simulink model "STM32Nucleo_VL53L1A1"  (R2023a)
settings: Solver=FixedStepDiscrete  StartTime=0.0  StopTime=inf  FixedStep=0.01  RelTol=1e-3  EnableMultiTasking=on
libraries: instrumentseriallib x3, nucleoutilitieslib x3, stmutilitieslib x3
settings Model: SimulationMode=external  PacingRate=0.100000  ExtModeTrigDuration=10  Creator=JesseJabezArendse  LastModifiedBy=JesseJabezArendse
settings OptimizationCC: ReuseModelBlockBuffer=off  PassReuseOutputArgsAs=Individual arguments  ZeroExternalMemoryAtStartup=off  ZeroInternalMemoryAtStartup=off  MaxStackSize=64  OptimizationLevel=level1  OptimizationCustomize=off  EfficientTunableParamExpr=on
settings DebuggingCC: ParameterPrecisionLossMsg=none  ParameterTunabilityLossMsg=error
settings HardwareCC: ProdBitPerPointer=32  ProdBitPerSizeT=32  ProdBitPerPtrDiffT=32  ProdLargestAtomicInteger=Long  ProdLargestAtomicFloat=Double  ProdWordSize=32  ProdLongLongMode=on  ProdHWDeviceType=ARM Compatible->ARM Cortex
settings ModelReferenceCC: EnableParallelModelReferenceBuilds=on
settings SFSimCC: SimCustomHeaderCode="#include \"Core\\Inc\\main.h\""  SimParseCustomCode=off  MATLABDynamicMemAlloc=off  SimHardwareAcceleration=native
settings SFSimCC: SimUserSources=|
  | Core\Src\main.c
  | Core\Src\IKS02A1_Simulink.c
settings SFSimCC: SimUserIncludeDirs=|
  | Core\Inc\
  | Core\Src\
settings RTWCC: Description=Embedded Coder  SystemTargetFile=ert.tlc  HardwareBoard=STM32 Nucleo F411RE  TemplateMakefile=ert_default_tmf  RTWUseSimCustomCode=on  CustomHeaderCode="#include \"Core\\Inc\\main.h\""  Toolchain=GNU Tools for ARM Embedded Processors  BuildConfiguration=Specify
settings RTWCC: CustomInclude=|
  | Core\Inc\
  | Core\Src\
settings RTWCC: CustomSource=|
  | Core\Src\main.c
  | Core\Src\IKS02A1_Simulink.c
settings CodeAppCC: ForceParamTrailComments=on  IgnoreCustomStorageClasses=off  OperatorAnnotations=on  SimulinkDataObjDesc=on  SFDataObjDesc=on  InsertBlockDesc=on
settings ERTTargetCC: CodeReplacementLibrary=ARM Cortex-M  SupportContinuousTime=on  ExtModeTransport=3  ExtModeStaticAlloc=on  ExtModeStaticAllocSize=2000  ExtModeMexFile=ext_xcp  ExtModeIntrfLevel=Level2 - Open

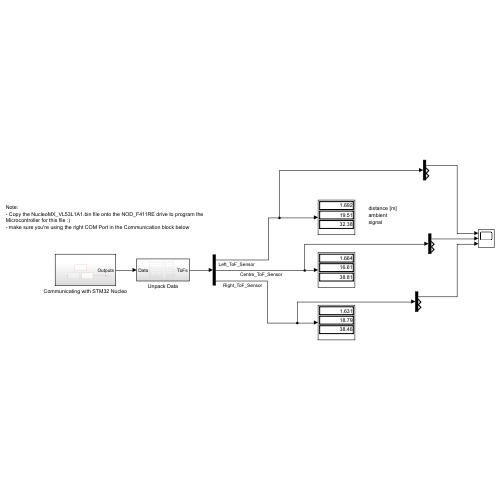
[thumbnail: Simulink's stored preview of the top-level diagram]
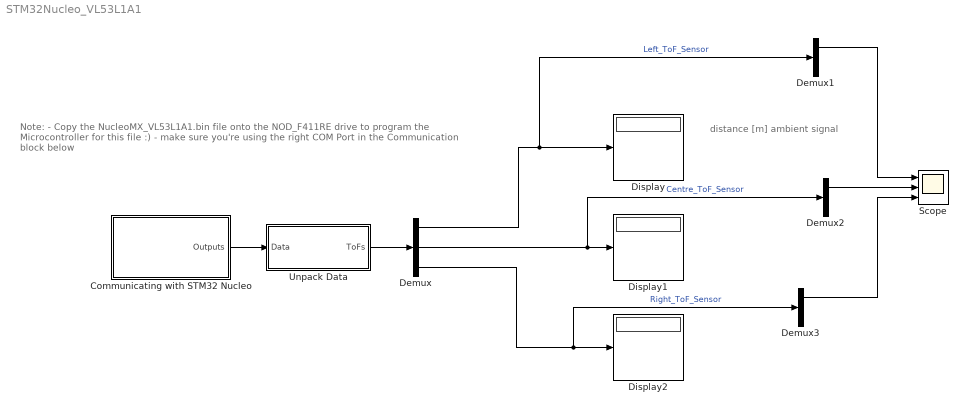
== system STM32Nucleo_VL53L1A1 ==
  note: distance [m]
      | ambient
      | signal
  note: Note:
      | - Copy the NucleoMX_VL53L1A1.bin file onto the NOD_F411RE drive to program the Microcontroller for this file :)
      | - make sure you're using the right COM Port in the Communication block below
  Communicating with STM32 Nucleo : Subsystem
  Demux : Demux  Outputs=[3 3 3]
  Demux1 : Demux  Outputs=3
  Demux2 : Demux  Outputs=3
  Demux3 : Demux  Outputs=3
  Display : Display
  Display1 : Display
  Display2 : Display
  Scope : Scope  NumInputPorts=3
  Unpack Data : Subsystem
  wires:
  Unpack Data/1(ToFs) -> Demux/1
  Demux/1 -> Demux1/1, Display/1  "Left_ToF_Sensor"
  Demux/2 -> Demux2/1, Display1/1  "Centre_ToF_Sensor"
  Demux/3 -> Demux3/1, Display2/1  "Right_ToF_Sensor"
  Communicating with STM32 Nucleo/1(Outputs) -> Unpack Data/1(Data)
  Demux1/1 -> Scope/1
  Demux2/1 -> Scope/2
  Demux3/1 -> Scope/3

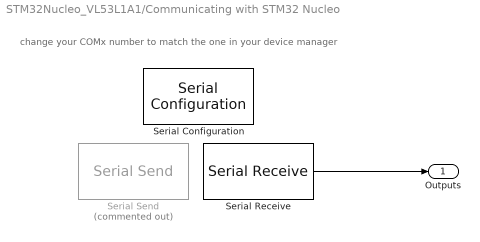
== system STM32Nucleo_VL53L1A1/Communicating with STM32 Nucleo ==
  note: change your COMx number to match the one in your device manager
  Serial Configuration : instrumentseriallib/Serial Configuration  Priority=-200000  PortSel=COM5  Port=COM5  ComPort=COM5  BaudRate=38400  DataBits=8  Parity=none  StopBits=1  ByteOrder=little-endian  FlowControl=none  Timeout=10  SimulateUsing=Interpreted execution  BlockInModel=on  aMode=1
      settings: LibrarySourceBlock=embeddedtargetslib/Host Communication/Serial Configuration
  Serial Receive : instrumentseriallib/Serial Receive  Priority=1  PortSel=COM5  Port=COM5  ComPort=COM5  DataType=single  SaveDataType=uint8  ToggleHeader=on  Header='J_A'  ToggleTerminator=on  Terminator=Custom terminator  CustomTerminator='A_J'  InputFormat=Column major  ToggleDataSize=on  DataSize=[1 9]  EnableBlockingMode=on  ActionDataUnavailable=Output last received value  ActionWhenDataUnavailable=Output last received value  CustomValue=0  SampleTime=-1  SimulateUsing=Interpreted execution  BlockInModel=on  aMode=1
      settings: LibrarySourceBlock=embeddedtargetslib/Host Communication/Serial Receive
  Serial Send : instrumentseriallib/Serial Send  Priority=1  Commented=on  PortSel=COM5  Port=COM5  ComPort=COM5  Header='J_A'  Terminator=Custom terminator  CustomTerminator='A_J'  EnableBlockingMode=on  SimulateUsing=Interpreted execution  BlockInModel=on  aMode=1
      settings: LibrarySourceBlock=embeddedtargetslib/Host Communication/Serial Send
  Outputs : Outport
  wires:
  Serial Receive/1 -> Outputs/1

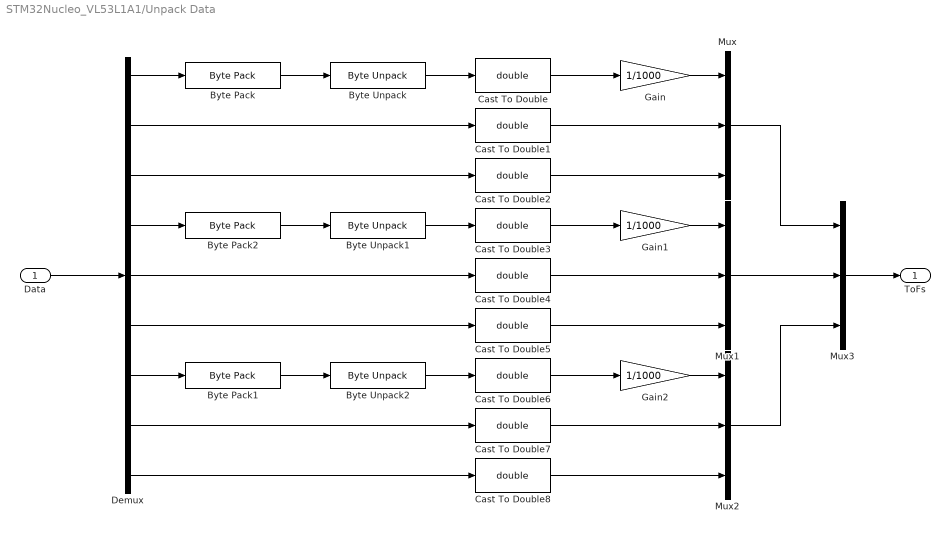
== system STM32Nucleo_VL53L1A1/Unpack Data ==
  Data : Inport
  Byte Pack : nucleoutilitieslib/Byte Pack  datatypes={'single'}  byteAlign=1  blockPlatform=nucleo
  Byte Pack1 : nucleoutilitieslib/Byte Pack  datatypes={'single'}  byteAlign=1  blockPlatform=nucleo
  Byte Pack2 : nucleoutilitieslib/Byte Pack  datatypes={'single'}  byteAlign=1  blockPlatform=nucleo
  Byte Unpack : stmutilitieslib/Byte Unpack  dimensions={[1]}  datatypes={'uint32'}  byteAlign=1  blockPlatform=stm32f4discovery
  Byte Unpack1 : stmutilitieslib/Byte Unpack  dimensions={[1]}  datatypes={'uint32'}  byteAlign=1  blockPlatform=stm32f4discovery
  Byte Unpack2 : stmutilitieslib/Byte Unpack  dimensions={[1]}  datatypes={'uint32'}  byteAlign=1  blockPlatform=stm32f4discovery
  Cast To Double{,1..8} (9 alike) : DataTypeConversion  OutDataTypeStr=double  SaturateOnIntegerOverflow=off  RndMeth=Floor
  Demux : Demux  Outputs=9
  Gain : Gain  Gain=1/1000
  Gain1 : Gain  Gain=1/1000
  Gain2 : Gain  Gain=1/1000
  Mux : Mux  Inputs=3
  Mux1 : Mux  Inputs=3
  Mux2 : Mux  Inputs=3
  Mux3 : Mux  Inputs=[3 3 3]
  ToFs : Outport
  wires:
  Mux3/1 -> ToFs/1
  Demux/7 -> Byte Pack1/1
  Cast To Double7/1 -> Mux2/2
  Demux/1 -> Byte Pack/1
  Demux/9 -> Cast To Double8/1
  Byte Unpack2/1 -> Cast To Double6/1
  Cast To Double1/1 -> Mux/2
  Byte Pack/1 -> Byte Unpack/1
  Cast To Double8/1 -> Mux2/3
  Demux/5 -> Cast To Double4/1
  Demux/6 -> Cast To Double5/1
  Byte Unpack/1 -> Cast To Double/1
  Demux/8 -> Cast To Double7/1
  Cast To Double2/1 -> Mux/3
  Mux2/1 -> Mux3/3
  Mux/1 -> Mux3/1
  Byte Pack1/1 -> Byte Unpack2/1
  Byte Unpack1/1 -> Cast To Double3/1
  Cast To Double/1 -> Gain/1
  Demux/2 -> Cast To Double1/1
  Byte Pack2/1 -> Byte Unpack1/1
  Demux/3 -> Cast To Double2/1
  Cast To Double5/1 -> Mux1/3
  Cast To Double3/1 -> Gain1/1
  Cast To Double4/1 -> Mux1/2
  Cast To Double6/1 -> Gain2/1
  Mux1/1 -> Mux3/2
  Demux/4 -> Byte Pack2/1
  Data/1 -> Demux/1
  Gain/1 -> Mux/1
  Gain1/1 -> Mux1/1
  Gain2/1 -> Mux2/1
